simulink model "gaintable"  (R2020b)
settings: Solver=FixedStepAuto  StartTime=0.0  StopTime=stop_time  RelTol=1e-3
values from neighbouring files (symbols this model uses):
  num_bands = 8    [gaintable_sim_init.m]
  prelookup_table_size = 24    [gaintable_sim_init.m]
  vy = [vy zeros(1,256-length(vy))]    [gaintable_sim_init.m]
  X_high = dB_max-dB_step    [gaintable_sim_init.m]
libraries: hdlsllib x2, simulink x1
settings Model: Creator=t96f346  LastModifiedBy=wickh
settings DataIOCC: SaveOutput=off  SaveTime=off  ReturnWorkspaceOutputs=off
settings OptimizationCC: BlockReduction=off  DefaultParameterBehavior=Inlined
settings ModelReferenceCC: ModelReferenceNumInstancesAllowed=Single

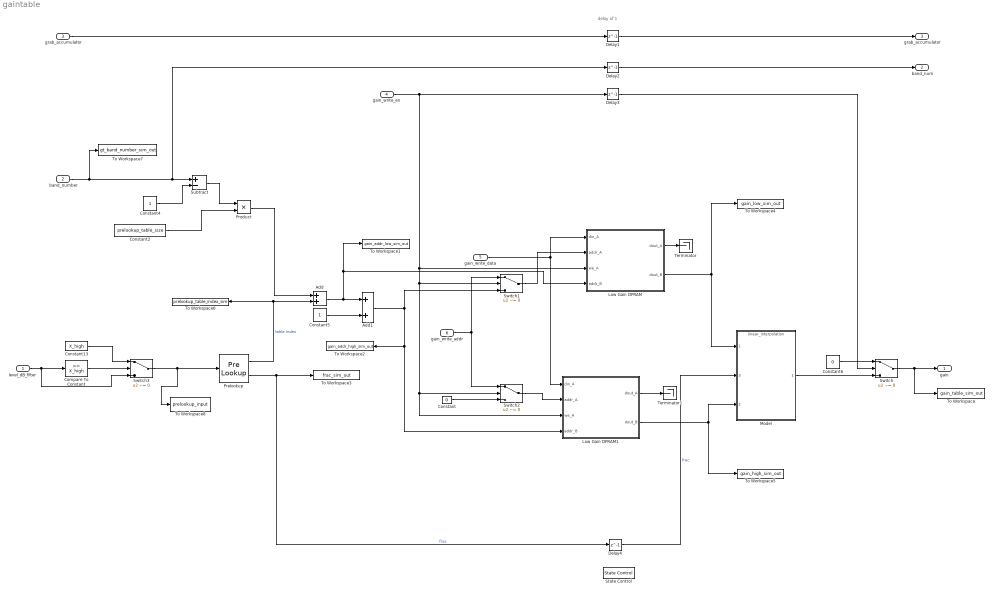
== system gaintable ==
  note: delay of 1
  level_dB_filter : Inport  OutDataTypeStr=input_type  PortDimensions=1
  band_number : Inport  Port=2  OutDataTypeStr=uint8  PortDimensions=1
  grab_accumulator : Inport  Port=3  OutDataTypeStr=boolean  PortDimensions=1
  gain_write_en : Inport  Port=4  OutDataTypeStr=boolean  PortDimensions=[1 1]
  gain_write_data : Inport  Port=5  OutDataTypeStr=gain_coeff_type  PortDimensions=[1 1]
  gain_write_addr : Inport  Port=6  OutDataTypeStr=uint8  PortDimensions=[1 1]
  Add : Sum  OutDataTypeStr=uint8
  Add1 : Sum  OutDataTypeStr=uint8
  Compare To Constant : simulink/Logic and Bit Operations/Compare To Constant  relop=>=  const=X_high  OutDataTypeStr=boolean
  Constant : Constant  Value=0  OutDataTypeStr=uint8  SampleTime=-1
  Constant13 : Constant  Value=X_high  OutDataTypeStr=input_type  SampleTime=-1
  Constant2 : Constant  Value=prelookup_table_size  OutDataTypeStr=uint8  SampleTime=-1
  Constant4 : Constant  OutDataTypeStr=uint8  SampleTime=-1
  Constant5 : Constant  OutDataTypeStr=uint8  SampleTime=-1
  Constant6 : Constant  Value=0  OutDataTypeStr=fixdt(1,16,8)  SampleTime=-1
  Delay{1..4} (4 alike) : Delay  DelayLength=1  InitialCondition=0
  Low Gain DPRAM : Subsystem
  Low Gain DPRAM1 : Subsystem
  Model : ModelReference  ModelNameDialog=linear_interpolation.slx  SimulationMode=Normal  ModelReferenceVersion=1.7
      settings: PortSchema="{\"entries\":[{\"content\":{\"sides\":[{\"content\":{\"connectorIds\":[\"In1\",\"In3\",\"In2\"]},\"type\":\"ConnectorPlacement.EquallySpacedRectSide\",\"uuid\":\"a1e49c79-2e82-4b14-9f86-0bba5ac5f1b9\"},{\"content\":{\"connectorIds\":[\"Out1\"],\"side\":\"RIGHT\"},\"type\":\"ConnectorPlacement.EquallySpacedRectSide\",\"uuid\":\"304d4c86-ec8b-4eb3-8394-1bee1e644227\"},{\"content\":{\"connectorIds\":[],\"side\":\"TOP\"},\"type\":\"ConnectorPlacement.EquallySpacedRectSide\",\"uuid\":\"baeac6e6-e190-4350-8c23-8e298d750d81\"},{\"content\":{\"connectorIds\":[],\"side\":\"HIDDEN\"},\"type\":\"ConnectorPlacement.EquallySpacedRectSide\",\"uuid\":\"d67e6ca1-e0bf-4e34-aac2-2b28a9a6e7dd\"}]},\"type\":\"ConnectorPlacement.EquallySpacedConnector\",\"uuid\":\"f761674e-d891-4606-80fe-18a36fbb3ba9\"}],\"packageUris\":[\"http://schema.mathworks.com/mf0/Connector/R2020b\"],\"version\":\"1.0\"}"
  Prelookup : PreLookup  BreakpointsData=input_levels_db  IndexSearchMethod=Evenly spaced points  UseLastBreakpoint=on  IndexDataTypeStr=uint8  RndMeth=Nearest
  Product : Product  OutDataTypeStr=Inherit: Same as first input
  State Control : StateControl  StateControl=Synchronous
  Subtract : Sum  Inputs=+-
  Switch : Switch  Criteria=u2 ~= 0  OutDataTypeStr=fixdt(1,16,8)
  Switch1 : Switch  Criteria=u2 ~= 0
  Switch2 : Switch  Criteria=u2 ~= 0
  Switch3 : Switch  Criteria=u2 ~= 0
  Terminator : Terminator
  Terminator1 : Terminator
  To Workspace : ToWorkspace  VariableName=gain_table_sim_out  SampleTime=-1
  To Workspace1 : ToWorkspace  VariableName=gain_addr_low_sim_out  SampleTime=-1
  To Workspace2 : ToWorkspace  VariableName=gain_addr_high_sim_out  SampleTime=-1
  To Workspace3 : ToWorkspace  VariableName=frac_sim_out  SampleTime=-1
  To Workspace4 : ToWorkspace  VariableName=gain_low_sim_out  SampleTime=-1
  To Workspace5 : ToWorkspace  VariableName=gain_high_sim_out  SampleTime=-1
  To Workspace6 : ToWorkspace  VariableName=prelookup_table_index_sim  SampleTime=-1
  To Workspace7 : ToWorkspace  VariableName=gt_band_number_sim_out  SampleTime=-1
  To Workspace8 : ToWorkspace  VariableName=prelookup_input  SampleTime=-1
  gain : Outport  OutDataTypeStr=gain_coeff_type  PortDimensions=[1 1]
  "band_num " : Outport  Port=2  PortDimensions=1
  "grab_accumulator " : Outport  Port=3  PortDimensions=1
  wires:
  Low Gain DPRAM1/2(dout_B) -> To Workspace5/1, Model/2
  Constant/1 -> Switch2/3
  Switch2/1 -> Low Gain DPRAM1/2(addr_A)
  Switch1/1 -> Low Gain DPRAM/2(addr_A)
  gain_write_addr/1 -> Switch1/1, Switch2/1
  gain_write_data/1 -> Low Gain DPRAM1/1(din_A), Low Gain DPRAM/1(din_A)
  Low Gain DPRAM1/1(dout_A) -> Terminator1/1
  Delay2/1 -> "band_num "/1
  Switch3/1 -> To Workspace8/1, Prelookup/1
  Constant2/1 -> Product/2
  level_dB_filter/1 -> Compare To Constant/1, Switch3/3
  Subtract/1 -> Product/1
  Product/1 -> Add/1
  Prelookup/2 -> Delay4/1, To Workspace3/1  "frac"
  Constant4/1 -> Subtract/2
  Low Gain DPRAM/2(dout_B) -> Model/1, To Workspace4/1
  Add1/1 -> Switch1/3, Low Gain DPRAM1/4(addr_B), To Workspace2/1
  Constant13/1 -> Switch3/1
  Prelookup/1 -> To Workspace6/1, Add/2  "table index"
  Constant5/1 -> Add1/2
  gain_write_en/1 -> Delay3/1, Switch2/2, Low Gain DPRAM1/3(we_A), Switch1/2, Low Gain DPRAM/3(we_A)
  Model/1 -> Switch/3
  Add/1 -> To Workspace1/1, Low Gain DPRAM/4(addr_B), Add1/1
  band_number/1 -> To Workspace7/1, Delay2/1, Subtract/1
  Switch/1 -> To Workspace/1, gain/1
  Compare To Constant/1 -> Switch3/2
  Delay3/1 -> Switch/2
  Delay4/1 -> Model/3  "frac"
  Constant6/1 -> Switch/1
  grab_accumulator/1 -> Delay1/1
  Delay1/1 -> "grab_accumulator "/1
  Low Gain DPRAM/1(dout_A) -> Terminator/1

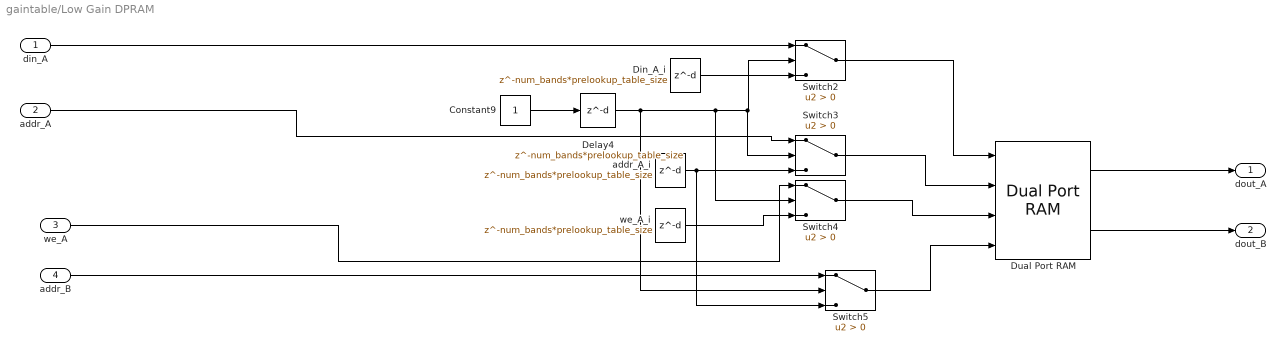
== system gaintable/Low Gain DPRAM ==
  din_A : Inport
  addr_A : Inport  Port=2
  we_A : Inport  Port=3
  addr_B : Inport  Port=4
  Constant9 : Constant  OutDataTypeStr=fixdt(0,16,16)  SampleTime=-1
  Delay4 : Delay  DelayLength=num_bands*prelookup_table_size  InitialCondition=0
  Din_A_i : Delay  DelayLength=num_bands*prelookup_table_size  InitialCondition=vy(1:num_bands*prelookup_table_size)
  Dual Port RAM : hdlsllib/HDL RAMs/Dual Port RAM  ram_size=8
      settings: SourceProductBaseCode=SL
  Switch{2..5} (4 alike) : Switch  Criteria=u2 > Threshold
  addr_A_i : Delay  DelayLength=num_bands*prelookup_table_size  InitialCondition=[0:(num_bands*prelookup_table_size- 1)]
  we_A_i : Delay  DelayLength=num_bands*prelookup_table_size  InitialCondition=1
  dout_A : Outport
  dout_B : Outport  Port=2  VectorParamsAs1DForOutWhenUnconnected=off
  wires:
  addr_A_i/1 -> Switch5/3, Switch3/3
  Switch2/1 -> Dual Port RAM/1
  Switch5/1 -> Dual Port RAM/4
  addr_A/1 -> Switch3/1
  Delay4/1 -> Switch5/2, Switch4/2, Switch3/2, Switch2/2
  Constant9/1 -> Delay4/1
  we_A_i/1 -> Switch4/3
  Switch3/1 -> Dual Port RAM/2
  Dual Port RAM/2 -> dout_B/1
  Switch4/1 -> Dual Port RAM/3
  din_A/1 -> Switch2/1
  Din_A_i/1 -> Switch2/3
  addr_B/1 -> Switch5/1
  we_A/1 -> Switch4/1
  Dual Port RAM/1 -> dout_A/1

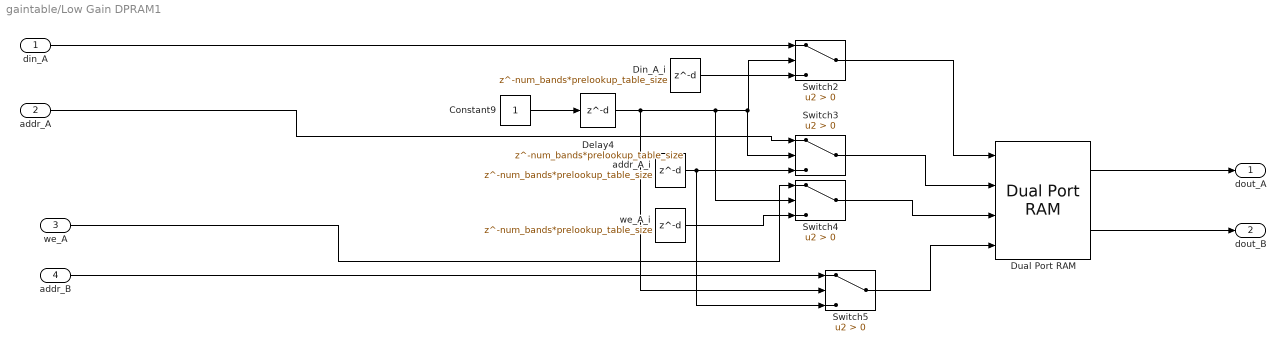
== system gaintable/Low Gain DPRAM1 ==
  din_A : Inport
  addr_A : Inport  Port=2
  we_A : Inport  Port=3
  addr_B : Inport  Port=4
  Constant9 : Constant  OutDataTypeStr=fixdt(0,16,16)  SampleTime=-1
  Delay4 : Delay  DelayLength=num_bands*prelookup_table_size  InitialCondition=0
  Din_A_i : Delay  DelayLength=num_bands*prelookup_table_size  InitialCondition=vy(1:num_bands*prelookup_table_size)
  Dual Port RAM : hdlsllib/HDL RAMs/Dual Port RAM  ram_size=8
      settings: SourceProductBaseCode=SL
  Switch{2..5} (4 alike) : Switch  Criteria=u2 > Threshold
  addr_A_i : Delay  DelayLength=num_bands*prelookup_table_size  InitialCondition=[0:(num_bands*prelookup_table_size- 1)]
  we_A_i : Delay  DelayLength=num_bands*prelookup_table_size  InitialCondition=1
  dout_A : Outport
  dout_B : Outport  Port=2  VectorParamsAs1DForOutWhenUnconnected=off
  wires:
  addr_A_i/1 -> Switch5/3, Switch3/3
  Switch2/1 -> Dual Port RAM/1
  Switch5/1 -> Dual Port RAM/4
  addr_A/1 -> Switch3/1
  Delay4/1 -> Switch5/2, Switch4/2, Switch3/2, Switch2/2
  Constant9/1 -> Delay4/1
  we_A_i/1 -> Switch4/3
  Switch3/1 -> Dual Port RAM/2
  Dual Port RAM/2 -> dout_B/1
  Switch4/1 -> Dual Port RAM/3
  din_A/1 -> Switch2/1
  Din_A_i/1 -> Switch2/3
  addr_B/1 -> Switch5/1
  we_A/1 -> Switch4/1
  Dual Port RAM/1 -> dout_A/1
